simulink model "Assignment_9"  (R2020b)
settings: Solver=VariableStepAuto  StartTime=0.0  StopTime=0.2  RelTol=1e-3
settings Model: Creator=Shantam Garg  LastModifiedBy=Shantam Garg

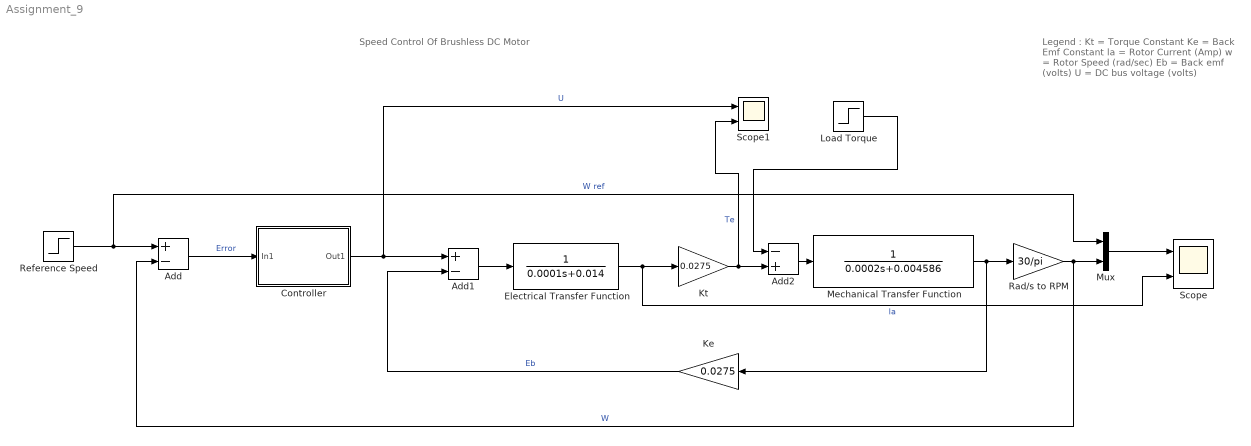
== system Assignment_9 ==
  note: Legend :
      | Kt = Torque Constant
      | Ke = Back Emf Constant
      | la = Rotor Current (Amp)
      | w = Rotor Speed (rad/sec)
      | Eb = Back emf (volts)
      | U = DC bus voltage (volts)
  note: Speed Control Of Brushless DC Motor
  Add : Sum  Inputs=+-
  Add1 : Sum  Inputs=+-
  Add2 : Sum  Inputs=-+
  Controller : Subsystem
  Electrical Transfer Function : TransferFcn  Denominator=[0.0001 0.014]
  Ke : Gain  Gain=0.0275
  Kt : Gain  Gain=0.0275
  Load Torque : Step  Time=0.1  After=10  SampleTime=0
  Mechanical Transfer Function : TransferFcn  Denominator=[0.0002 0.004586]
  Mux : Mux  Inputs=2
  Rad/s to RPM : Gain  Gain=30/pi
  Reference Speed : Step  Time=0  After=1500  SampleTime=0
  Scope : Scope  NumInputPorts=2
  Scope1 : Scope  NumInputPorts=2
  wires:
  Reference Speed/1 -> Add/1, Mux/1  "W ref"
  Add1/1 -> Electrical Transfer Function/1
  Electrical Transfer Function/1 -> Scope/2, Kt/1  "la"
  Kt/1 -> Add2/2, Scope1/2  "Te"
  Add2/1 -> Mechanical Transfer Function/1
  Mechanical Transfer Function/1 -> Ke/1, Rad/s to RPM/1
  Rad/s to RPM/1 -> Mux/2, Add/2  "W"
  Load Torque/1 -> Add2/1
  Ke/1 -> Add1/2  "Eb"
  Mux/1 -> Scope/1
  Controller/1(Out1) -> Add1/1, Scope1/1  "U"
  Add/1 -> Controller/1(In1)  "Error"

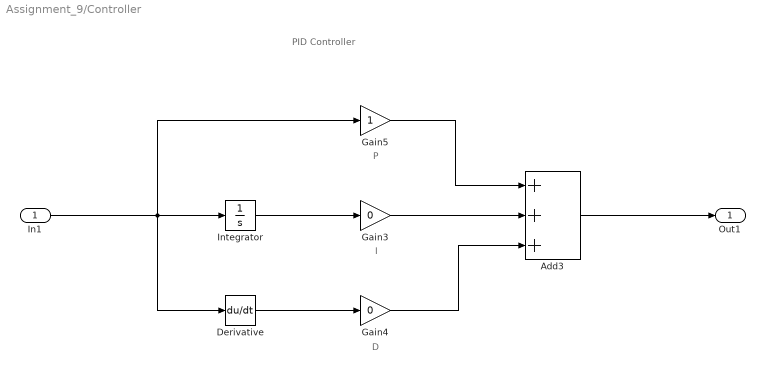
== system Assignment_9/Controller ==
  note: PID Controller
  note: P
  note: I
  note: D
  In1 : Inport
  Add3 : Sum  Inputs=+++
  Derivative : Derivative
  Gain3 : Gain  Gain=0
  Gain4 : Gain  Gain=0
  Gain5 : Gain
  Integrator : Integrator
  Out1 : Outport
  wires:
  Add3/1 -> Out1/1
  Integrator/1 -> Gain3/1
  Gain3/1 -> Add3/2
  Gain5/1 -> Add3/1
  Derivative/1 -> Gain4/1
  Gain4/1 -> Add3/3
  In1/1 -> Derivative/1, Gain5/1, Integrator/1
